simulink model "discreteHopfieldNetwork"  (R2017a)
settings: Solver=FixedStepAuto  StartTime=0.0  StopTime=10.0  FixedStep=1  RelTol=1e-3  EnableMultiTasking=on
undefined symbols (not defined in the file or in its folder): ib, T, v0
settings Model: Creator=Lucas  LastModifiedBy=Lucas
settings OptimizationCC: LifeSpan=inf
settings DebuggingCC: SFUnexpectedBacktrackingDiag=warning  SFNoUnconditionalDefaultTransitionDiag=warning  SFExecutionAtInitializationDiag=none
settings GRTTargetCC: TargetLangStandard=C89/C90 (ANSI)  GeneratePreprocessorConditionals=Disable all
settings ConfigComp: CovMetricSettings=dw  CovHtmlReporting=on  CovSaveCumulativeToWorkspaceVar=on  CovSaveSingleToWorkspaceVar=on  CovExternalEMLEnable=off

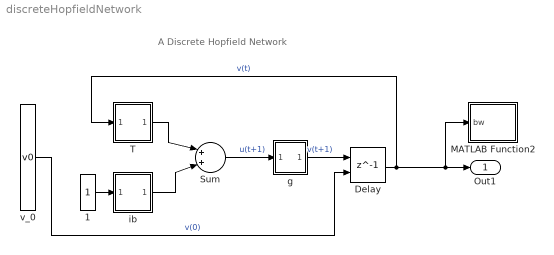
== system discreteHopfieldNetwork ==
  note: A Discrete Hopfield Network
  1 : Constant
      mask Display: disp('1')
  Delay : Delay  DelayLength=1  InitialConditionSource=Input port  SampleTime=1
      settings: InputPortMap=u0,p4
  MATLAB Function2 : MATLAB Function  TreatAsAtomicUnit=on
  Sum : Sum  Inputs=|++|
  T : Subsystem
      mask Display: disp('T')
  g : Subsystem
      mask Display:
      | plot([-1 1]*0.35+0.5,[0 0]+0.15)
      | plot([-1 0 0 1]*0.35+0.5,[-1 -1 1 1]*0.35+0.5);
      | %plot([0 1 1 0 0],[0 0 1 1 0]);
  ib : Subsystem
      mask Display: disp('i^b')
  v_0 : Constant  Value=v0
      mask Display: disp('')
  Out1 : Outport
  wires:
  v_0/1 -> Delay/2  "v(0)"
  Delay/1 -> MATLAB Function2/1(bw), Out1/1, T/1(In1)  "v(t)"
  T/1(Out1) -> Sum/1
  Sum/1 -> g/1(In1)  "u(t+1)"
  g/1(Out1) -> Delay/1  "v(t+1)"
  1/1 -> ib/1(In1)
  ib/1(Out1) -> Sum/2

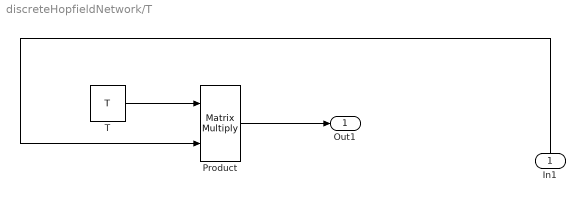
== system discreteHopfieldNetwork/T ==
  In1 : Inport
  Product : Product  Multiplication=Matrix(*)
  T : Constant  Value=T
  Out1 : Outport
  wires:
  In1/1 -> Product/2
  T/1 -> Product/1
  Product/1 -> Out1/1

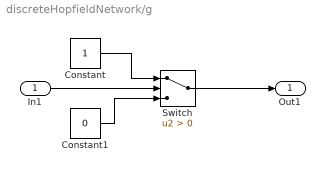
== system discreteHopfieldNetwork/g ==
  In1 : Inport
  Constant : Constant
  Constant1 : Constant  Value=0
  Switch : Switch  Criteria=u2 > Threshold
  Out1 : Outport
  wires:
  In1/1 -> Switch/2
  Switch/1 -> Out1/1
  Constant/1 -> Switch/1
  Constant1/1 -> Switch/3

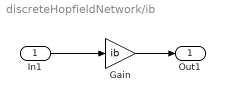
== system discreteHopfieldNetwork/ib ==
  In1 : Inport
  Gain : Gain  Gain=ib
  Out1 : Outport
  wires:
  Gain/1 -> Out1/1
  In1/1 -> Gain/1

== matlab function discreteHopfieldNetwork/MATLAB Function2 ==
  data: bw input
function plot(bw)
coder.extrinsic('imshow')
bw = reshape(bw, 6, 5);

xh = [0.5000; 5.5000; 5.5000; 0.5000; 0.5000; 5.5000; 5.5000; 0.5000; 0.5000; 5.5000; 5.5000; 0.5000; 0.5000; 5.5000];
yh = [0.5000; 0.5000; 1.5000; 1.5000; 2.5000; 2.5000; 3.5000; 3.5000; 4.5000; 4.5000; 5.5000; 5.5000; 6.5000; 6.5000];

xv = [0.5000; 0.5000; 1.5000; 1.5000; 2.5000; 2.5000; 3.5000; 3.5000; 4.5000; 4.5000; 5.5000; 5.5000];
yv = [0.5000; 6.5000; 6.5000; 0.5000; 0.5000; 6.5000; 6.5000; 0.5000; 0.5000; 6.5000; 6.5000; 0.5000];

h = imshow(ones(size(bw)) - bw, 'InitialMagnification', 'fit');
ax = ancestor(h, 'axes');
line('Parent', ax, 'XData', xh, 'YData', yh, ...
    'Color', 'r', 'LineWidth', 2, 'Clipping', 'off');
line('Parent', ax, 'XData', xv, 'YData', yv, ...
    'Color', 'r', 'LineWidth', 2, 'Clipping', 'off');
